simulink model "TV_2017_HIL"  (R2016a)
settings: Solver=ode1  StartTime=0.0  StopTime=600  FixedStep=0.001  RelTol=1e-3
PreLoadFcn:
  | HIL_parameters
values from neighbouring files (symbols this model uses):
  battery_voltage = single(530)    [HIL_parameters.m]    (also in HIL_parameters_2018.m; TV_2017_parameters.m; TV_2017_parameters_VD.m)
  car_params = Simulink_Car_params    [HIL_parameters.m]    (also in HIL_parameters_2018.m; TV_2017_parameters.m; TV_2017_parameters_VD.m)
  i_Diff = 16    [HIL_parameters.m]    (also in HIL_parameters_2018.m; TV_2017_parameters.m)
  Kp = 1    [HIL_parameters.m]    (also in HIL_parameters_2018.m; TV_2017_parameters.m; TV_2017_parameters_VD.m)
  motor_data = struct    [HIL_parameters.m]    (also in HIL_parameters_2018.m; TV_2017_parameters.m)
  settings = Simulink_Settings    [HIL_parameters.m]    (also in HIL_parameters_2018.m; TV_2017_parameters.m; TV_2017_parameters_VD.m)
  SpdC_BCC = 0    [HIL_parameters.m]    (also in HIL_parameters_2018.m; TV_2017_parameters.m; TV_2017_parameters_VD.m)
  Speed_Neg_sat = -21    [HIL_parameters.m]    (also in HIL_parameters_2018.m; TV_2017_parameters.m; TV_2017_parameters_VD.m)
  Speed_Pos_sat = 21    [HIL_parameters.m]    (also in HIL_parameters_2018.m; TV_2017_parameters.m; TV_2017_parameters_VD.m)
  SteeringAngleFL = [-23.80 -22.65 -21.50 -20.34 -19.18 -18.03 -16.86 -15.70 -14.53 -13.35 -12.18 -10.99 -9.80 -8.61 -7.40 -6.19 -4.97 -3.75 -2.51 -1.26 0 1.27 2.56 3.85 5.17 6.50 7.84 9.21 10.59 12.00 13.42 14.88 16.36 17.87 19.41 20.99 22.61 24.26 25.97 27.73 29.54]    [CarSetupAnalysis2018.m]    (also in HIL_parameters_2018.m; TV_2017_parameters.m; TV_2017_parameters_VD.m = [-24.129 -22.950 -21.772 -20.593 -19.413 -18.232 -17.050 -15)
  SteeringAngleFR = [-29.54 -27.73 -25.97 -24.26 -22.61 -20.99 -19.41 -17.87 -16.36 -14.88 -13.42 -12.00 -10.59 -9.21 -7.84 -6.50 -5.17 -3.85 -2.56 -1.27 0 1.26 2.51 3.75 4.97 6.19 7.40 8.61 9.80 10.99 12.18 13.35 14.53 15.70 16.86 18.03 19.18 20.34 21.50 22.65 23.80]    [CarSetupAnalysis2018.m]    (also in HIL_parameters_2018.m; TV_2017_parameters.m; TV_2017_parameters_VD.m = [-29.3050 -27.5340 -25.8140 -24.1410 -22.5110 -20.9180 -19.3)
  SteeringWhAngle = [-105 -99.75 -94.5 -89.25 -84 -78.75 -73.5 -68.25 -63 -57.75 -52.5 -47.25 -42 -36.75 -31.5 -26.25 -21.0 -15.75 -10.5 -5.25 0.0 5.25 10.50 15.75 21.00 26.25 31.50 36.75 42.00 47.25 52.50 57.75  63.00 68.25 73.50 78.75 84.00 89.25 94.50 99.75 105.00]    [TV_2017_parameters_VD.m]
  Tn_n = 0    [HIL_parameters.m]    (also in HIL_parameters_2018.m; TV_2017_parameters.m; TV_2017_parameters_VD.m)
  Use_Joystick = 1    [HIL_parameters.m]    (also in HIL_parameters_2018.m; TV_2017_parameters.m; TV_2017_parameters_VD.m)
undefined symbols (not defined in the file or in its folder): canChannel, TC_Decr_Gas, TC_Derivative, TC_Incr_Gas, TC_On, TC_Relay_Off, TC_Relay_On
libraries: CarMaker4SL x314, canmsglib x48, simulink_extras x48, simulink x41, canlib x39, powerlib_meascontrol x2, sldrtlib x1
(part 1 of 9)
settings Model: Creator=fh  LastModifiedBy=95fre
settings SolverCC: EnableConcurrentExecution=on  InsertRTBMode=Always
settings DataIOCC: LimitDataPoints=on  SaveFormat=Array  SignalLoggingSaveFormat=ModelDataLogs  SignalLoggingName=sigsOut
settings OptimizationCC: BlockReduction=off  OptimizeBlockIOStorage=off  BufferReuse=off  GlobalBufferReuse=off  ExpressionFolding=off  ExpressionDepthLimit=2147483647  LocalBlockOutputs=off  InitFltsAndDblsToZero=on
settings DebuggingCC: SaveWithParameterizedLinksMsg=none  UnderspecifiedInitializationDetection=Classic  MergeDetectMultiDrivingBlocksExec=none  SignalResolutionControl=TryResolveAllWithWarning  MultiTaskDSMMsg=warning  MultiTaskCondExecSysMsg=none  FcnCallInpInsideContextMsg=UseLocalSettings  BusObjectLabelMismatch=error  StateNameClashWarn=warning
settings HardwareCC: ProdBitPerLong=64  ProdLargestAtomicFloat=None  ProdHWDeviceType=Intel->x86-64  TargetBitPerLong=64  TargetBitPerPointer=64  TargetIntDivRoundTo=Zero  TargetEndianess=LittleEndian  TargetWordSize=64  TargetHWDeviceType=Intel->x86-64
settings ModelReferenceCC: PropagateSignalLabelsOutOfModel=off
settings SFSimCC: SimCtrlC=off
settings RTWCC: SystemTargetFile=sldrt.tlc  TemplateMakefile=sldrt.tmf  Description=Simulink Desktop Real-Time  Toolchain=LCC-win64 v2.4.1 | gmake (64-bit Windows)  BuildConfiguration=Faster Runs  RTWCompilerOptimization=on  CheckMdlBeforeBuild=Warning
settings CodeAppCC: MaxIdLength=95
settings SimulinkDesktopRealTimeCC: TargetPreCompLibLocation=C:\Program Files\MATLAB\R2016a\toolbox\sldrt\lib\win64  TargetLangStandard=C89/C90 (ANSI)  SupportVariableSizeSignals=off
settings ConfigComp: CovModelRefEnable=Off

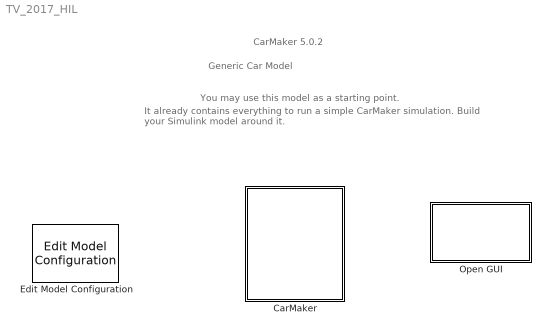
== system TV_2017_HIL ==
  note: Generic Car Model
  note: You may use this model as a starting point.
  note: It already contains everything to run a simple CarMaker simulation.
      | Build your Simulink model around it.
  note: CarMaker 5.0.2
  CarMaker : Subsystem  TreatAsAtomicUnit=on
      mask Display: image(imread('CarMaker4SLss.bmp'));
  Edit Model Configuration : CarMaker4SL/Edit Model Configuration
  Open GUI : Subsystem  LoadFcn=if ~length(which('cmcmd')), cmenv; end
      settings: OpenFcn=cmblockmagic('gui_fix_display'); CM_Simulink
      mask Display: image(imread('CarMakerGUI.bmp'));

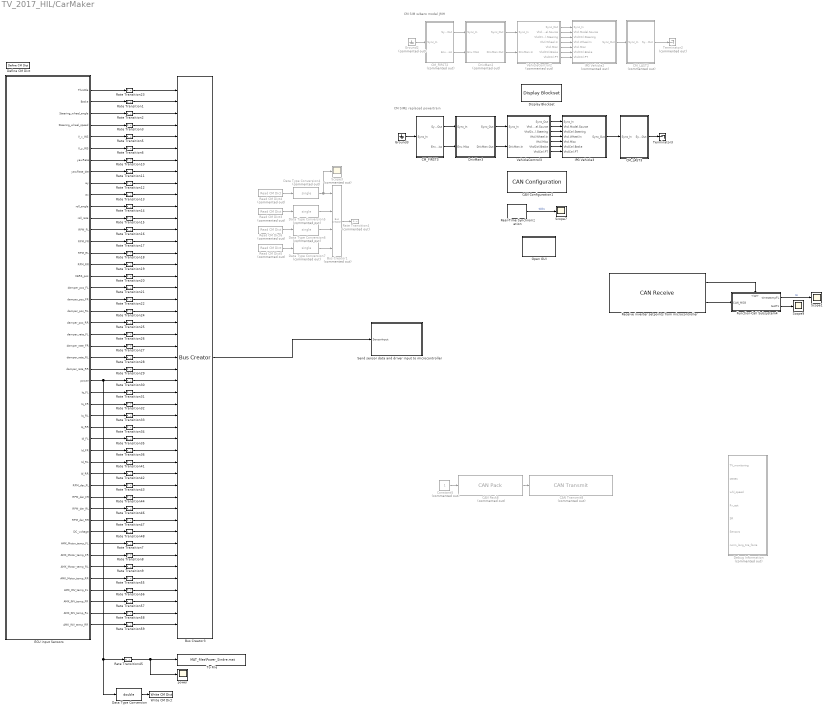
== system TV_2017_HIL/CarMaker ==
  note: CM SIM w/Aero model JMH
  note: CM SIM|| replaced powertrain
  Bus Creator1 : BusCreator  Commented=on  Inputs=4  OutDataTypeStr=Bus: normalForces  NonVirtualBus=on
      settings: InheritFromInputs=off
  Bus Creator3 : BusCreator  Inputs=47  OutDataTypeStr=Bus: SensorInputs  NonVirtualBus=on
      settings: InheritFromInputs=off
  CAN Configuration1 : canlib/CAN Configuration  BlockHandle=8130.0005  DeviceMenu=(none)  Device=PEAK-System PCAN-PCI Express (PCAN_PCIBUS1)  ObjConstructor=canChannel('PEAK-System', 'PCAN_PCIBUS1')  BusSpeed=1000000  EnableBitParameters=off  SJW=NaN  TSEG1=NaN  TSEG2=NaN  NSamples=NaN  AckMode=Normal
  CAN Pack8 : canmsglib/CAN Pack  Commented=on  MsgList=(none)  MsgName=CAN Msg  MsgIDType=Standard (11-bit identifier)  MsgIdentifier=5  MsgLength=1  SignalInfo=Signal1$0$8$1$1$1$0$1$0$-Inf$Inf$#  NSignals=1  StartBits=str2num('[int32(0)]')  SignalSizes=str2num('[int32(8)]')  ByteOrders=str2num('[int32(1)]')  DataTypes=str2num('[int32(1)]')  MultiplexTypes=str2num('[int32(1)]')  MultiplexValues=str2num('[double(0)]')  Factors=str2num('[double(1)]')  Offsets=str2num('[double(0)]')  Minimums=str2num('[double(-Inf)]')  Maximums=str2num('[double(Inf)]')  Remote=off
      settings: DataFormat=manually specified signals
  CAN Transmit8 : canlib/CAN Transmit  Commented=on  BlockHandle=8132.0005  DeviceMenu=(none)  Device=PEAK-System PCAN-PCI Express (PCAN_PCIBUS1)  ObjConstructor=canChannel('PEAK-System', 'PCAN_PCIBUS1')  EnablePeriodicTransmit=off  MessagePeriod=1.000
  CM_FIRST2 : Subsystem  Commented=on
  CM_FIRST3 : Subsystem
  CM_LAST2 : Subsystem  Commented=on
  CM_LAST3 : Subsystem
  Constant5 : Constant  Commented=on
  Data Type Conversion : DataTypeConversion  OutDataTypeStr=double
  Data Type Conversion{4..7} (4 alike) : DataTypeConversion  Commented=on  OutDataTypeStr=single
  "Debug Information " : Subsystem  Commented=on
  Define CM Dict : CarMaker4SL/Define CM Dict  xname=Power  xmono=off  xtype=Double  xdvaplace=None  xnstates=0  xfirststate=0  xinitial=0
  Display Blockset : CarMaker4SL/Display Blockset
  DrivMan2 : Subsystem  Commented=on
  DrivMan3 : Subsystem
  "ECU input Sensors " : Subsystem  SystemSampleTime=settings.control_system_sample_time
  Function-Call Subsystem4 : Subsystem  TreatAsAtomicUnit=on
  Ground2 : Ground  Commented=on
  Ground3 : Ground
  IPG Vehicle2 : Subsystem  Commented=on  TreatAsAtomicUnit=on
  IPG Vehicle3 : Subsystem  TreatAsAtomicUnit=on
  Open GUI : Subsystem  LoadFcn=if ~length(which('cmcmd')), cmenv; end
      settings: OpenFcn=cmblockmagic('gui_fix_display'); CM_Simulink
      mask Display: image(imread('CarMakerGUI.bmp'));
  Rate Transition{1..3,5..36,41..48,55..59} (48 alike) : RateTransition  OutPortSampleTime=matlab_params.sensor_sampling_time
  Rate Transition4 : RateTransition  Commented=on  OutPortSampleTime=settings.sensor_sampling_time
  Read CM Dict3 : CarMaker4SL/Read CM Dict  Commented=on  xname=Vhcl.FR.Fz  xsync=off
  Read CM Dict4 : CarMaker4SL/Read CM Dict  Commented=on  xname=Vhcl.FL.Fz  xsync=off
  Read CM Dict5 : CarMaker4SL/Read CM Dict  Commented=on  xname=Vhcl.RR.Fz  xsync=off
  Read CM Dict6 : CarMaker4SL/Read CM Dict  Commented=on  xname=Vhcl.RL.Fz  xsync=off
  Real-Time Synchronization : sldrtlib/Real-Time Synchronization  SampleTime=0.01  MaxMissedTicks=100000  ShowMissedTicks=on  YieldWhenWaiting=on
  Receive inverter setpoints from microcontroller : canlib/CAN Receive  BlockHandle=21848.0001  DeviceMenu=(none)  Device=PEAK-System PCAN-PCI Express (PCAN_PCIBUS1)  ObjConstructor=canChannel('PEAK-System', 'PCAN_PCIBUS1')  EnableStandardIDsFilter=off  StandardIDs=listen_ID  EnableExtendedIDsFilter=off  ExtendedIDs=0  SampleTime=0.001  MsgsPerTimestep=all  StdIDsCombo=Allow all  ExtIDsCombo=Block all  InternalFilterUpdateStatus=on
  Scope1 : Scope
  Scope3 : Scope  Commented=on
  Scope7 : Scope
  Scope9 : Scope
  "Send sensor data and driver input to microcontroller " : Subsystem
  Terminator2 : Terminator  Commented=on
  Terminator3 : Terminator
  To File : ToFile  Filename=MAT_files\Power_Sindre.mat  MatrixName=Power  SaveFormat=Timeseries
  VehicleControl2 : Subsystem  Commented=on
  VehicleControl3 : Subsystem
  Write CM Dict : CarMaker4SL/Write CM Dict  xname=Power  xsync=off
  power : Scope
  wires:
  Read CM Dict3/1 -> Data Type Conversion5/1
  Read CM Dict4/1 -> Data Type Conversion4/1
  Read CM Dict5/1 -> Data Type Conversion7/1
  Read CM Dict6/1 -> Data Type Conversion6/1
  Data Type Conversion6/1 -> Bus Creator1/3
  Data Type Conversion7/1 -> Bus Creator1/4
  Data Type Conversion5/1 -> Bus Creator1/2
  Data Type Conversion4/1 -> Scope3/1, Bus Creator1/1
  Bus Creator1/1 -> Rate Transition4/1
  Real-Time Synchronization/1 -> Scope7/1  "ticks"
  Receive inverter setpoints from microcontroller/2 -> Function-Call Subsystem4/1(CAN_MSG)
  Receive inverter setpoints from microcontroller/1 -> Function-Call Subsystem4/Trigger
  Function-Call Subsystem4/1(timestampFL) -> Scope1/1  "ts"
  Function-Call Subsystem4/2(testTs) -> Scope9/1
  ? -> ?
  CAN Pack8/1 -> CAN Transmit8/1
  Constant5/1 -> CAN Pack8/1
  CM_FIRST2/2(Env.Misc) -> DrivMan2/2(Env.Misc)
  VehicleControl2/2(Vhcl.Model.Source) -> IPG Vehicle2/2(Vhcl.Model.Source)
  VehicleControl2/6(VhclCtrl.Brake) -> IPG Vehicle2/6(VhclCtrl.Brake)
  VehicleControl2/3(VhclCtrl.Steering) -> IPG Vehicle2/3(VhclCtrl.Steering)
  DrivMan2/2(DrivMan.Out) -> VehicleControl2/2(DrivMan.In)
  CM_FIRST2/1(Sync_Out) -> DrivMan2/1(Sync_In)
  VehicleControl2/7(VhclCtrl.PT) -> IPG Vehicle2/7(VhclCtrl.PT)
  VehicleControl2/4(Vhcl.Wheel.In) -> IPG Vehicle2/4(Vhcl.Wheel.In)
  VehicleControl2/1(Sync_Out) -> IPG Vehicle2/1(Sync_In)
  IPG Vehicle2/1(Sync_Out) -> CM_LAST2/1(Sync_In)
  DrivMan2/1(Sync_Out) -> VehicleControl2/1(Sync_In)
  Ground2/1 -> CM_FIRST2/1(Sync_In)
  CM_LAST2/1(Sync_Out) -> Terminator2/1
  VehicleControl2/5(Vhcl.Misc) -> IPG Vehicle2/5(Vhcl.Misc)
  VehicleControl3/7(VhclCtrl.PT) -> IPG Vehicle3/7(VhclCtrl.PT)
  VehicleControl3/6(VhclCtrl.Brake) -> IPG Vehicle3/6(VhclCtrl.Brake)
  CM_FIRST3/1(Sync_Out) -> DrivMan3/1(Sync_In)
  CM_FIRST3/2(Env.Misc) -> DrivMan3/2(Env.Misc)
  VehicleControl3/3(VhclCtrl.Steering) -> IPG Vehicle3/3(VhclCtrl.Steering)
  DrivMan3/2(DrivMan.Out) -> VehicleControl3/2(DrivMan.In)
  VehicleControl3/2(Vhcl.Model.Source) -> IPG Vehicle3/2(Vhcl.Model.Source)
  VehicleControl3/5(Vhcl.Misc) -> IPG Vehicle3/5(Vhcl.Misc)
  VehicleControl3/1(Sync_Out) -> IPG Vehicle3/1(Sync_In)
  VehicleControl3/4(Vhcl.Wheel.In) -> IPG Vehicle3/4(Vhcl.Wheel.In)
  DrivMan3/1(Sync_Out) -> VehicleControl3/1(Sync_In)
  Ground3/1 -> CM_FIRST3/1(Sync_In)
  IPG Vehicle3/1(Sync_Out) -> CM_LAST3/1(Sync_In)
  CM_LAST3/1(Sync_Out) -> Terminator3/1
  Rate Transition45/1 -> power/1, To File/1
  "ECU input Sensors "/37(RPM_der_RL) -> Rate Transition46/1
  "ECU input Sensors "/38(RPM_der_RR) -> Rate Transition47/1
  "ECU input Sensors "/36(RPM_der_FR) -> Rate Transition44/1
  "ECU input Sensors "/35(RPM_der_FL) -> Rate Transition43/1
  "ECU input Sensors "/34(Id_RR) -> Rate Transition42/1
  "ECU input Sensors "/4(Steering_wheel_speed) -> Rate Transition3/1
  "ECU input Sensors "/1("Throttle ") -> Rate Transition23/1
  "ECU input Sensors "/2("Brake ") -> Rate Transition1/1
  "ECU input Sensors "/3("Steering_wheel_angle ") -> Rate Transition2/1
  "ECU input Sensors "/5(V_x_INS) -> Rate Transition5/1
  "ECU input Sensors "/6(V_y_INS) -> Rate Transition6/1
  "ECU input Sensors "/7(yawRate) -> Rate Transition10/1
  "ECU input Sensors "/9(ay) -> Rate Transition12/1
  "ECU input Sensors "/10("ax ") -> Rate Transition13/1
  "ECU input Sensors "/11(roll_angle) -> Rate Transition14/1
  "ECU input Sensors "/12(roll_rate) -> Rate Transition15/1
  "ECU input Sensors "/13(RPM_FL) -> Rate Transition16/1
  "ECU input Sensors "/14(RPM_FR) -> Rate Transition17/1
  "ECU input Sensors "/15(RPM_RL) -> Rate Transition18/1
  "ECU input Sensors "/16(RPM_RR) -> Rate Transition19/1
  "ECU input Sensors "/17(KERS_pos) -> Rate Transition20/1
  "ECU input Sensors "/18(damper_pos_FL) -> Rate Transition21/1
  "ECU input Sensors "/19(damper_pos_FR) -> Rate Transition22/1
  "ECU input Sensors "/20(damper_pos_RL) -> Rate Transition24/1
  "ECU input Sensors "/21(damper_pos_RR) -> Rate Transition25/1
  "ECU input Sensors "/22(damper_rate_FL) -> Rate Transition26/1
  "ECU input Sensors "/23(damper_rate_FR) -> Rate Transition27/1
  "ECU input Sensors "/24(damper_rate_RL) -> Rate Transition28/1
  "ECU input Sensors "/25(damper_rate_RR) -> Rate Transition29/1
  "ECU input Sensors "/27(Iq_FL) -> Rate Transition31/1
  "ECU input Sensors "/28(Iq_FR) -> Rate Transition32/1
  "ECU input Sensors "/29(Iq_RL) -> Rate Transition33/1
  "ECU input Sensors "/30(Iq_RR) -> Rate Transition34/1
  "ECU input Sensors "/31(Id_FL) -> Rate Transition35/1
  "ECU input Sensors "/32(Id_FR) -> Rate Transition36/1
  "ECU input Sensors "/33(Id_RL) -> Rate Transition41/1
  "ECU input Sensors "/8(yawRate_der) -> Rate Transition11/1
  "ECU input Sensors "/39(DC_voltage) -> Rate Transition48/1
  Rate Transition23/1 -> Bus Creator3/1
  Rate Transition17/1 -> Bus Creator3/14
  Rate Transition12/1 -> Bus Creator3/9
  Rate Transition30/1 -> Bus Creator3/26
  Rate Transition14/1 -> Bus Creator3/11
  Rate Transition16/1 -> Bus Creator3/13
  Rate Transition25/1 -> Bus Creator3/21
  Rate Transition3/1 -> Bus Creator3/4
  Rate Transition2/1 -> Bus Creator3/3
  Rate Transition22/1 -> Bus Creator3/19
  Rate Transition11/1 -> Bus Creator3/8
  Rate Transition18/1 -> Bus Creator3/15
  Rate Transition20/1 -> Bus Creator3/17
  Rate Transition1/1 -> Bus Creator3/2
  Rate Transition24/1 -> Bus Creator3/20
  Rate Transition31/1 -> Bus Creator3/27
  Rate Transition26/1 -> Bus Creator3/22
  Rate Transition29/1 -> Bus Creator3/25
  Rate Transition15/1 -> Bus Creator3/12
  Rate Transition13/1 -> Bus Creator3/10
  Rate Transition28/1 -> Bus Creator3/24
  Rate Transition19/1 -> Bus Creator3/16
  Rate Transition21/1 -> Bus Creator3/18
  Rate Transition27/1 -> Bus Creator3/23
  Rate Transition5/1 -> Bus Creator3/5
  Rate Transition6/1 -> Bus Creator3/6
  Rate Transition42/1 -> Bus Creator3/34
  Rate Transition47/1 -> Bus Creator3/38
  Rate Transition48/1 -> Bus Creator3/39
  Rate Transition41/1 -> Bus Creator3/33
  Rate Transition43/1 -> Bus Creator3/35
  Rate Transition35/1 -> Bus Creator3/31
  Rate Transition34/1 -> Bus Creator3/30
  Rate Transition46/1 -> Bus Creator3/37
  Rate Transition44/1 -> Bus Creator3/36
  Rate Transition33/1 -> Bus Creator3/29
  Rate Transition32/1 -> Bus Creator3/28
  Rate Transition36/1 -> Bus Creator3/32
  Rate Transition10/1 -> Bus Creator3/7
  "ECU input Sensors "/26(power) -> Data Type Conversion/1, Rate Transition45/1, Rate Transition30/1
  Data Type Conversion/1 -> Write CM Dict/1
  "ECU input Sensors "/44(AMK_INV_temp_FL) -> Rate Transition56/1
  "ECU input Sensors "/40(AMK_Motor_temp_FL) -> Rate Transition7/1
  "ECU input Sensors "/41(AMK_Motor_temp_FR) -> Rate Transition8/1
  "ECU input Sensors "/42(AMK_Motor_temp_RL) -> Rate Transition9/1
  "ECU input Sensors "/43(AMK_Motor_temp_RR) -> Rate Transition55/1
  "ECU input Sensors "/45(AMK_INV_temp_FR) -> Rate Transition57/1
  "ECU input Sensors "/46(AMK_INV_temp_RL) -> Rate Transition58/1
  "ECU input Sensors "/47(AMK_INV_temp_RR) -> Rate Transition59/1
  Rate Transition7/1 -> Bus Creator3/40
  Rate Transition8/1 -> Bus Creator3/41
  Rate Transition9/1 -> Bus Creator3/42
  Rate Transition55/1 -> Bus Creator3/43
  Rate Transition56/1 -> Bus Creator3/44
  Rate Transition57/1 -> Bus Creator3/45
  Rate Transition58/1 -> Bus Creator3/46
  Rate Transition59/1 -> Bus Creator3/47
  Bus Creator3/1 -> "Send sensor data and driver input to microcontroller "/1(SensorInput)

== system TV_2017_HIL/Open GUI ==
  S-Function : S-Function  FunctionName=cm_gui  SFunctionDeploymentMode=off  EnableBusSupport=off

== system TV_2017_HIL/CarMaker/CM_FIRST2 ==
  Sync_In : Inport
  Bus Creator1 : BusCreator  Inputs=9
  Demux : Demux  Outputs=9
  Environment : S-Function  FunctionName=CM_Sfun  Parameters='Environment'  SFunctionDeploymentMode=off  EnableBusSupport=off
  IoIn : S-Function  FunctionName=CM_Sfun  Parameters='IoIn'  SFunctionDeploymentMode=off  EnableBusSupport=off
  Sync_Out : Outport
  Env.Misc : Outport  Port=2
  wires:
  Bus Creator1/1 -> Env.Misc/1
  Environment/2 -> Demux/1
  Demux/4 -> Bus Creator1/4  "Env AirHumidity"
  Demux/3 -> Bus Creator1/3  "Env AirPressure"
  Demux/2 -> Bus Creator1/2  "Env AirDensity"
  Demux/1 -> Bus Creator1/1  "Env Temperature"
  Environment/1 -> Sync_Out/1
  IoIn/1 -> Environment/1
  Sync_In/1 -> IoIn/1
  Demux/5 -> Bus Creator1/5  "Env Time"
  Demux/6 -> Bus Creator1/6  "Env SolarRadiation"
  Demux/7 -> Bus Creator1/7  "Env WindVel_tot x"
  Demux/8 -> Bus Creator1/8  "Env WindVel_tot y"
  Demux/9 -> Bus Creator1/9  "Env WindVel_tot z"

== system TV_2017_HIL/CarMaker/CM_FIRST3 ==
  Sync_In : Inport
  BusCreator1 : BusCreator  Inputs=8
  BusCreator2 : BusCreator  Inputs=6
  Demux1 : Demux  Outputs=14
  Environment : S-Function  FunctionName=CM_Sfun  Parameters='Environment'  SFunctionDeploymentMode=off  EnableBusSupport=off
  IoIn : S-Function  FunctionName=CM_Sfun  Parameters='IoIn'  SFunctionDeploymentMode=off  EnableBusSupport=off
  Terminator : Terminator
  Sync_Out : Outport
  Env.Misc : Outport  Port=2
  wires:
  BusCreator2/1 -> Terminator/1  "IF Environment (in)"
  BusCreator1/1 -> Env.Misc/1
  Demux1/14 -> BusCreator2/6  "Env sRoad"
  Demux1/13 -> BusCreator2/5  "Env PoI_GCS Elev"
  Demux1/12 -> BusCreator2/4  "Env PoI_GCS Lat"
  Demux1/11 -> BusCreator2/3  "Env PoI_GCS Long"
  Demux1/10 -> BusCreator2/2  "Env Time"
  Demux1/9 -> BusCreator2/1  "Env yDay"
  Demux1/8 -> BusCreator1/8  "Env WindVel_tot z"
  Demux1/7 -> BusCreator1/7  "Env WindVel_tot y"
  Demux1/6 -> BusCreator1/6  "Env WindVel_tot x"
  Demux1/5 -> BusCreator1/5  "Env SolarRadiation"
  Demux1/4 -> BusCreator1/4  "Env AirHumidity"
  Demux1/3 -> BusCreator1/3  "Env AirPressure"
  Demux1/2 -> BusCreator1/2  "Env AirDensity"
  Demux1/1 -> BusCreator1/1  "Env Temperature"
  Environment/2 -> Demux1/1
  Environment/1 -> Sync_Out/1
  IoIn/1 -> Environment/1
  Sync_In/1 -> IoIn/1

== system TV_2017_HIL/CarMaker/CM_LAST2 ==
  Sync_In : Inport
  CM_User : S-Function  FunctionName=CM_Sfun  Parameters='CM_User'  SFunctionDeploymentMode=off  EnableBusSupport=off
  IoOut : S-Function  FunctionName=CM_Sfun  Parameters='IoOut'  SFunctionDeploymentMode=off  EnableBusSupport=off
  Sync_Out : Outport
  wires:
  IoOut/1 -> Sync_Out/1
  CM_User/1 -> IoOut/1
  Sync_In/1 -> CM_User/1

== system TV_2017_HIL/CarMaker/CM_LAST3 ==
  Sync_In : Inport
  CM_User : S-Function  FunctionName=CM_Sfun  Parameters='CM_User'  SFunctionDeploymentMode=off  EnableBusSupport=off
  IoOut : S-Function  FunctionName=CM_Sfun  Parameters='IoOut'  SFunctionDeploymentMode=off  EnableBusSupport=off
  Sync_Out : Outport
  wires:
  IoOut/1 -> Sync_Out/1
  CM_User/1 -> IoOut/1
  Sync_In/1 -> CM_User/1

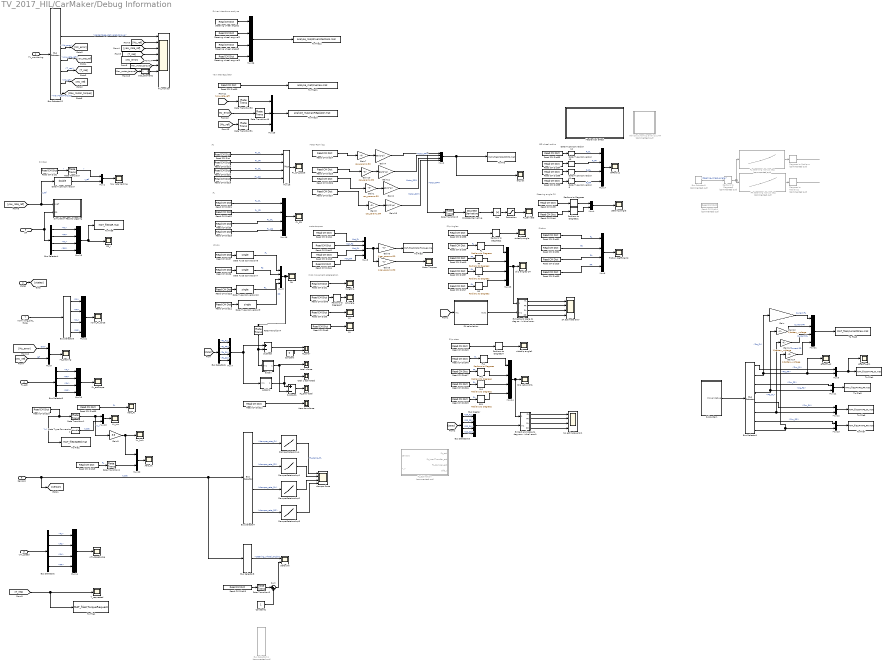
== system TV_2017_HIL/CarMaker/Debug Information  ==
  note: SimRes
  note: Eff wheel radius
  note: motortorques
  note: Friction
  note: FZ CM
  note: Fy
  note: FX
  note: misc movement acceleration
  note: Steering angle CM
  note: Motor Rpm log
  note: Slip Angles
  note: Slip rates
  note: Yaw rate regulator
  note: Driver intentions analyze
  TV_monitoring : Inport
  states : Inport  Port=2
  whl_speed : Inport  Port=3
  Fx_est : Inport  Port=4
  "SR " : Inport  Port=5
  Sensors : Inport  Port=6
  norm_long_tire_force : Inport  Port=7
  Abs : Abs
  "Aero downforce " : Scope
  Aero_Fx : Scope
  Aero_Fz : Scope
  Bus Creator : BusCreator  Inputs=4
  Bus Selector1 : BusSelector  OutputSignals=Pm_FL,Pe_FL,Pm_FR,Pe_FR,Pm_RL,Pe_RL,Pm_RR,Pe_RR
  Bus Selector10 : BusSelector  OutputSignals=SR_FL,SR_FR,SR_RL,SR_RR
  Bus Selector11 : BusSelector  Commented=on  OutputSignals=steering_wheel_angle
  Bus Selector12 : BusSelector  OutputSignals=active_contraints,saturated_constraints,percentage_delivered_torque,Mz_error,yaw_rate_ref,T_req,Mz_ref,maxMotorTorque
  Bus Selector{2..5} (4 alike) : BusSelector  OutputSignals=FL,FR,RL,RR
  Bus Selector6 : BusSelector  OutputSignals=Fz_FL,Fz_FR,Fz_RL,Fz_RR
  Bus Selector7 : BusSelector  OutputSignals=damper_rate_FL,damper_rate_FR,damper_rate_RL,damper_rate_RR
  Bus Selector8 : BusSelector  OutputSignals=steering_wheel_angle
  Bus Selector9 : BusSelector  Commented=on  OutputSignals=steering_wheel_angle
  Constant : Constant  Value=0
  Constant1 : Constant
  DamperRateLookup : Lookup_n-D  NumberOfTableDimensions=1  BreakpointsForDimension1=car_params.damper_table_breakpoint;  Table=car_params.damper_pull_push_values_front;  ExtrapMethod=Clip  UseLastTableValue=on  InternalRulePriority=Speed  RndMeth=Simplest  InputSameDT=on
  DamperRateLookup1 : Lookup_n-D  NumberOfTableDimensions=1  BreakpointsForDimension1=car_params.damper_table_breakpoint;  Table=car_params.damper_pull_push_values_front;  ExtrapMethod=Clip  UseLastTableValue=on  InternalRulePriority=Speed  RndMeth=Simplest  InputSameDT=on
  DamperRateLookup2 : Lookup_n-D  NumberOfTableDimensions=1  BreakpointsForDimension1=car_params.damper_table_breakpoint;  Table=car_params.damper_pull_push_values_rear;  ExtrapMethod=Clip  UseLastTableValue=on  InternalRulePriority=Speed  RndMeth=Simplest  InputSameDT=on
  DamperRateLookup3 : Lookup_n-D  NumberOfTableDimensions=1  BreakpointsForDimension1=car_params.damper_table_breakpoint;  Table=car_params.damper_pull_push_values_rear;  ExtrapMethod=Clip  UseLastTableValue=on  InternalRulePriority=Speed  RndMeth=Simplest  InputSameDT=on
  Data Type Conversion : DataTypeConversion  OutDataTypeStr=double
  Data Type Conversion1 : DataTypeConversion  OutDataTypeStr=double
  Data Type Conversion{6..13} (8 alike) : DataTypeConversion  OutDataTypeStr=single
  Degrees to Radians : simulink_extras/Transformations/Degrees to Radians  Commented=on
  Degrees to Radians1 : simulink_extras/Transformations/Degrees to Radians  Commented=on
  Discrete Derivative : simulink/Discrete/Discrete Derivative  gainval=1.0  ICPrevScaledInput=0.0  InputProcessing=Inherited  OutMin=[]  OutMax=[]  OutDataType=fixdt(1, 16)  OutScaling=2^-10  DoSatur=off
  Extract and scale to deg compare to CM output in individual error : Subsystem
  Extract and scale to deg compare to CM output in individual error1 : Subsystem
  FL : simulink_extras/Transformations/Radians to Degrees
  FL steer ang lookup deg : Lookup_n-D  Commented=on  NumberOfTableDimensions=1  BreakpointsForDimension1=SteeringWhAngle  Table=SteeringAngleFL  ExtrapMethod=Clip  UseLastTableValue=on  InternalRulePriority=Speed  RndMeth=Simplest  InputSameDT=on
  FL1 : simulink_extras/Transformations/Radians to Degrees
  FR : simulink_extras/Transformations/Radians to Degrees
  FR steer ang lookup deg : Lookup_n-D  Commented=on  NumberOfTableDimensions=1  BreakpointsForDimension1=SteeringWhAngle  Table=SteeringAngleFR  ExtrapMethod=Clip  UseLastTableValue=on  InternalRulePriority=Speed  RndMeth=Simplest  InputSameDT=on
  FR1 : simulink_extras/Transformations/Radians to Degrees
  FY_CM : Scope
  Fl_derivate : Scope
  Fx_CM_scope : Scope
  Fx_estScope : Scope
  Fz_Estimation : Subsystem  Commented=on  TreatAsAtomicUnit=on
  Fz_error : Scope  NumInputPorts=2
  Fz_error total : Scope
  Fzi : Scope
  Gain{,12..14} (4 alike) : Gain  Gain=1/battery_voltage
  Gain{1,3,7,10} (4 alike) : Gain  Gain=car_params.GR
  Gain{2,4,11,15} (4 alike) : Gain  Gain=60/(2*pi)
  Gain5 : Gain  Gain=1/car_params.GR
  Gain6 : Gain  Gain=1/car_params.GR
  Gain9 : Gain  Gain=3.6
  Mechanical effect : Subsystem
  "Motor Torques " : Scope
  Mux{1,4..5,9..13,20} (9 alike) : Mux  Inputs=2
  Mux{2..3,6..8,14..19,21..24,26} (16 alike) : Mux
  Mux25 : Mux  Inputs=3
  Mz_tracking : Scope
  RL : simulink_extras/Transformations/Radians to Degrees
  RL1 : simulink_extras/Transformations/Radians to Degrees
  RR : simulink_extras/Transformations/Radians to Degrees
  RR1 : simulink_extras/Transformations/Radians to Degrees
  Radians to Degrees{,1..2,4,7} (5 alike) : simulink_extras/Transformations/Radians to Degrees
  Radians to Degrees3 : simulink_extras/Transformations/Radians to Degrees  Commented=on
  Rate Transition{,1..5} (6 alike) : RateTransition  OutPortSampleTime=matlab_params.control_system_sample_time
  Rate Transition49 : RateTransition  OutPortSampleTimeOpt=Inherit
  Rate Transition50 : RateTransition  OutPortSampleTimeOpt=Inherit
  Rate Transition51 : RateTransition  OutPortSampleTimeOpt=Inherit
  Read CM Dict : CarMaker4SL/Read CM Dict  xname=Vhcl.FL.Fx  xsync=off
  Read CM Dict1 : CarMaker4SL/Read CM Dict  xname=Car.LongSlipRL  xsync=off
  Read CM Dict10 : CarMaker4SL/Read CM Dict  xname=Car.vx  xsync=off
  Read CM Dict11 : CarMaker4SL/Read CM Dict  xname=Vhcl.RR.Fz  xsync=off
  Read CM Dict12 : CarMaker4SL/Read CM Dict  xname=Car.Aero.Frc_1.z  xsync=off
  Read CM Dict13 : CarMaker4SL/Read CM Dict  xname=Vhcl.Steer.Ang  xsync=off
  Read CM Dict14 : CarMaker4SL/Read CM Dict  Commented=on  xsync=off
  Read CM Dict15 : CarMaker4SL/Read CM Dict  xname=Car.LongSlipRR  xsync=off
  Read CM Dict16 : CarMaker4SL/Read CM Dict  xname=Car.LongSlipRL  xsync=off
  Read CM Dict17 : CarMaker4SL/Read CM Dict  xname=Car.SlipAngleRR  xsync=off
  Read CM Dict18 : CarMaker4SL/Read CM Dict  xname=Vhcl.FR.Fx  xsync=off
  Read CM Dict19 : CarMaker4SL/Read CM Dict  xname=Vhcl.RR.Fx  xsync=off
  Read CM Dict2 : CarMaker4SL/Read CM Dict  xname=Car.YawRate  xsync=off
  Read CM Dict20 : CarMaker4SL/Read CM Dict  xname=Vhcl.RL.Fx  xsync=off
  Read CM Dict21 : CarMaker4SL/Read CM Dict  xname=Vhcl.FL.Fy  xsync=off
  Read CM Dict22 : CarMaker4SL/Read CM Dict  xname=Vhcl.FR.Fy  xsync=off
  Read CM Dict23 : CarMaker4SL/Read CM Dict  xname=Vhcl.RR.Fy  xsync=off
  Read CM Dict24 : CarMaker4SL/Read CM Dict  xname=Car.WheelSpd_FL  xsync=off
  Read CM Dict25 : CarMaker4SL/Read CM Dict  xname=Car.WheelSpd_FR  xsync=off
  Read CM Dict26 : CarMaker4SL/Read CM Dict  xname=Car.WheelSpd_RL  xsync=off
  Read CM Dict27 : CarMaker4SL/Read CM Dict  xname=Car.WheelSpd_RR  xsync=off
  Read CM Dict28 : CarMaker4SL/Read CM Dict  xname=Vhcl.RL.Fz  xsync=off
  Read CM Dict29 : CarMaker4SL/Read CM Dict  xname=Car.muRoadRL  xsync=off
  Read CM Dict3 : CarMaker4SL/Read CM Dict  xname=Car.CFR.rz  xsync=off
  Read CM Dict30 : CarMaker4SL/Read CM Dict  xname=Car.muRoadRR  xsync=off
  Read CM Dict31 : CarMaker4SL/Read CM Dict  xname=Car.muRoadFL  xsync=off
  Read CM Dict32 : CarMaker4SL/Read CM Dict  xname=Car.muRoadFR  xsync=off
  Read CM Dict33 : CarMaker4SL/Read CM Dict  xname=Car.WFL.Radius  xsync=off
  Read CM Dict34 : CarMaker4SL/Read CM Dict  xname=Car.WFR.Radius  xsync=off
  Read CM Dict35 : CarMaker4SL/Read CM Dict  xname=Car.WRR.Radius  xsync=off
  Read CM Dict36 : CarMaker4SL/Read CM Dict  xname=Car.WRL.Radius  xsync=off
  Read CM Dict37 : CarMaker4SL/Read CM Dict  xname=Car.SlipAngleRL  xsync=off
  Read CM Dict38 : CarMaker4SL/Read CM Dict  xname=Car.SideSlipAngle  xsync=off
  Read CM Dict39 : CarMaker4SL/Read CM Dict  xname=Car.SlipAngleFL  xsync=off
  Read CM Dict4 : CarMaker4SL/Read CM Dict  xname=Car.CFL.rz  xsync=off
  Read CM Dict40 : CarMaker4SL/Read CM Dict  xname=Car.SlipAngleFR  xsync=off
  Read CM Dict41 : CarMaker4SL/Read CM Dict  xname=PT.WFL.Trq_Drive  xsync=off
  Read CM Dict42 : CarMaker4SL/Read CM Dict  xname=PT.WFR.Trq_Drive  xsync=off
  Read CM Dict43 : CarMaker4SL/Read CM Dict  xname=PT.WRL.Trq_Drive  xsync=off
  Read CM Dict44 : CarMaker4SL/Read CM Dict  xname=PT.WRR.Trq_Drive  xsync=off
  Read CM Dict45 : CarMaker4SL/Read CM Dict  xname=Car.SideSlipAngle  xsync=off
  Read CM Dict46 : CarMaker4SL/Read CM Dict  xname=Car.LongSlipFL  xsync=off
  Read CM Dict47 : CarMaker4SL/Read CM Dict  xname=Car.LongSlipFR  xsync=off
  Read CM Dict48 : CarMaker4SL/Read CM Dict  xname=Vhcl.Roll  xsync=off
  Read CM Dict49 : CarMaker4SL/Read CM Dict  xname=Car.Aero.Frc_1.z  xsync=off
  Read CM Dict5 : CarMaker4SL/Read CM Dict  xname=Vhcl.RL.Fy  xsync=off
  Read CM Dict50 : CarMaker4SL/Read CM Dict  xname=Vhcl.YawRate  xsync=off
  Read CM Dict53 : CarMaker4SL/Read CM Dict  xname=Car.Aero.Frc_1.x  xsync=off
  Read CM Dict6 : CarMaker4SL/Read CM Dict  xname=Vhcl.FR.Fz  xsync=off
  Read CM Dict7 : CarMaker4SL/Read CM Dict  xname=Vhcl.FL.Fz  xsync=off
  Read CM Dict8 : CarMaker4SL/Read CM Dict  xname=Car.ax  xsync=off
  Read CM Dict9 : CarMaker4SL/Read CM Dict  xname=Car.ay  xsync=off
  SA calculation : Subsystem
  SA estimate error : Scope  NumInputPorts=4
  SA estimate error1 : Scope  NumInputPorts=4
  SR_i : Scope
  Saturation : Saturate  UpperLimit=50000
  Simulation Results Logging : Subsystem
  Slip angles CM : Scope
  Slip ratios CM1 : Scope
  Steering wheel ang-vel2 : CarMaker4SL/Read CM Dict  xname=DM.Steer.AngVel  xsync=off
  Steering wheel ang-vel3 : CarMaker4SL/Read CM Dict  xname=DM.Brake  xsync=off
  Steering wheel angle2 : CarMaker4SL/Read CM Dict  xname=DM.Steer.Ang  xsync=off
  Steering wheel angle3 : CarMaker4SL/Read CM Dict  xname=DM.Gas  xsync=off
  Subsystem : Subsystem
  Subtract : Sum  Inputs=+-
  Subtract1 : Sum  Inputs=+-
  Sum : Sum  Inputs=|++
  TV_monitor : Scope  NumInputPorts=9
  "T_requested " : Scope
  To File : ToFile  Filename=MAT_files\MotorRPMS.mat  MatrixName=MotorRpms  SaveFormat=Timeseries
  To File1 : ToFile  Filename=MAT_files\TorqueRequest  MatrixName=TorqueRequest  SaveFormat=Timeseries
  To File10 : ToFile  Filename=analyse_mat/yawRegulator.mat  MatrixName=yaw_reg  SaveFormat=Timeseries
  To File11 : ToFile  Filename=analyse_mat/trueYaw.mat  MatrixName=vhclYaw  SaveFormat=Timeseries
  To File12 : ToFile  Filename=analyse_mat/driverIntentions.mat  MatrixName=driverIntentions  SaveFormat=Timeseries
  To File2 : ToFile  Filename=MAT_files\Speed.mat  MatrixName=VehicleSpeed  SaveFormat=Timeseries
  To File3 : ToFile  Filename=MAT_files\MotorTorques.mat  MatrixName=MotorTorques  SaveFormat=Timeseries
  To File4 : ToFile  Filename=MAT_files\PmPe_FL.mat  MatrixName=PmPe_FL  SaveFormat=Timeseries
  To File5 : ToFile  Filename=MAT_files\PmPe_FR.mat  MatrixName=PmPe_FR  SaveFormat=Timeseries
  To File6 : ToFile  Filename=MAT_files\PmPe_RL.mat  MatrixName=PmPe_RL  SaveFormat=Timeseries
  To File7 : ToFile  Filename=MAT_files\PmPe_RR.mat  MatrixName=PmPe_RR  SaveFormat=Timeseries
  To File8 : ToFile  Filename=MAT_files\SR.mat  MatrixName=SR  SaveFormat=Timeseries
  To File9 : ToFile  Filename=MAT_files\currentDraw.mat  SaveFormat=Timeseries
  Vehicle dynamics analysis JMH : Subsystem  Commented=on
  Vx_kmh : Scope
  "Vx_ms " : Scope
  Yaw rate tracking : Scope
  add_elements : Subsystem
  addall : Subsystem
  addall1 : Subsystem
  ax : Scope
  ay : Scope
  damper force : Scope  NumInputPorts=4
  delta SW : Scope  NumInputPorts=2
  effRadius : Scope
  effectFL_el : Scope
  effectFL_el1 : Scope
  eng rot : Scope
  friction coefficients : Scope
  "longSlip " : Scope
  norm_Fx_force : Scope
  rollAngle : Scope
  sideslip angle : Scope
  sideslip angle1 : Scope
  steering angle : Scope
  total z estimated : Scope
  total z force : Scope
  whl_speed_cog : Scope
  wires:
  [T_req] -> To File1/1, "T_requested "/1
  [Mz_error] -> Mux9/1  "error"
  [Mz_ref] -> Mux9/2  "ref"
  Mux9/1 -> Mz_tracking/1
  Mux5/1 -> effectFL_el1/1, To File4/1
  Mux11/1 -> To File5/1
  Mux12/1 -> To File6/1
  Mux13/1 -> To File7/1
  Subsystem/1(Power debug) -> Bus Selector1/1
  Bus Selector1/1 -> Mux5/1  "<Pm_FL>"
  Bus Selector1/2 -> Gain/1, effectFL_el/1, Mux5/2  "<Pe_FL>"
  Bus Selector1/3 -> Mux11/1  "<Pm_FR>"
  Bus Selector1/4 -> Gain12/1, Mux11/2  "<Pe_FR>"
  Bus Selector1/5 -> Mux12/1  "<Pm_RL>"
  Bus Selector1/6 -> Gain13/1, Mux12/2  "<Pe_RL>"
  Bus Selector1/7 -> Mux13/1  "<Pm_RR>"
  Bus Selector1/8 -> Gain14/1, Mux13/2  "<Pe_RR>"
  whl_speed/1 -> Bus Selector2/1
  Bus Selector2/4 -> Mux14/4  "<RR>"
  Bus Selector2/3 -> Mux14/3  "<RL>"
  Bus Selector2/2 -> Mux14/2  "<FR>"
  Bus Selector2/1 -> Mux14/1  "<FL>"
  Mux14/1 -> whl_speed_cog/1
  Fx_est/1 -> Bus Selector3/1
  Bus Selector3/1 -> Mux15/1  "<FL>"
  Bus Selector3/2 -> Mux15/2  "<FR>"
  Bus Selector3/3 -> Mux15/3  "<RL>"
  Bus Selector3/4 -> Mux15/4  "<RR>"
  Mux15/1 -> Fx_estScope/1
  Read CM Dict53/1 -> Aero_Fx/1  "FL"
  Read CM Dict10/1 -> To File2/1, Rate Transition1/1  "V_x"
  Mux10/1 -> "Vx_ms "/1
  Rate Transition1/1 -> Gain9/1, Mux10/1  "V_x"
  Data Type Conversion1/1 -> Mux10/2  "V_est"
  Gain9/1 -> Mux20/1, Vx_kmh/1
  Mux20/1 -> Aero_Fz/1
  Read CM Dict49/1 -> Rate Transition2/1  "FL"
  Rate Transition2/1 -> Mux20/2
  Gain/1 -> Mux21/1  "Current FL"
  Gain12/1 -> Mux21/2  "Current FR"
  Gain13/1 -> Mux21/3  "Current RL"
  Gain14/1 -> Mux21/4  "Current RR"
  Mux21/1 -> To File9/1
  norm_long_tire_force/1 -> Bus Selector5/1
  Bus Selector5/1 -> Mux22/1  "<FL>"
  Bus Selector5/4 -> Mux22/4  "<RR>"
  Bus Selector5/3 -> Mux22/3  "<RL>"
  Bus Selector5/2 -> Mux22/2  "<FR>"
  Mux22/1 -> norm_Fx_force/1
  Rate Transition3/1 -> Discrete Derivative/1
  Saturation/1 -> Fl_derivate/1
  Abs/1 -> Saturation/1
  Discrete Derivative/1 -> Abs/1
  Mux2/1 -> eng rot/1, To File/1
  Read CM Dict27/1 -> Gain3/1
  Read CM Dict26/1 -> Gain1/1
  Gain15/1 -> Mux2/4  "Motor_RPM"
  Gain3/1 -> Gain15/1
  Gain2/1 -> Mux2/3  "Motor_RPM"
  Gain1/1 -> Gain2/1
  Gain11/1 -> Mux2/2  "Motor_RPM"
  Gain10/1 -> Gain11/1
  Read CM Dict25/1 -> Gain10/1
  Read CM Dict24/1 -> Gain7/1
  Gain4/1 -> Mux2/1, Rate Transition3/1  "Motor_RPM"
  Gain7/1 -> Gain4/1
  Radians to Degrees1/1 -> Mux4/2
  Mux4/1 -> steering angle/1
  Read CM Dict3/1 -> Radians to Degrees/1
  Read CM Dict4/1 -> Radians to Degrees1/1
  Radians to Degrees/1 -> Mux4/1
  Read CM Dict48/1 -> Radians to Degrees7/1
  Radians to Degrees7/1 -> rollAngle/1
  Read CM Dict9/1 -> ay/1
  Read CM Dict8/1 -> ax/1
  Read CM Dict1/1 -> "longSlip "/1
  Mux16/1 -> Fx_CM_scope/1
  Read CM Dict18/1 -> Mux16/2  "Fx_FR"
  Read CM Dict19/1 -> Mux16/4  "Fx_RR"
  Read CM Dict20/1 -> Mux16/3  "Fx_RL"
  Read CM Dict/1 -> Mux16/1  "Fx_FL"
  Mux18/1 -> FY_CM/1
  Read CM Dict22/1 -> Mux18/2  "Fy_FR"
  Read CM Dict5/1 -> Mux18/3  "Fy_RL"
  Read CM Dict23/1 -> Mux18/4  "Fy_RR"
  Read CM Dict21/1 -> Mux18/1  "Fy_FL"
  Data Type Conversion10/1 -> Mux3/3  "RL"
  Data Type Conversion7/1 -> Mux3/2  "FR"
  Mux3/1 -> Rate Transition4/1, Fzi/1
  Read CM Dict7/1 -> Data Type Conversion8/1
  Read CM Dict11/1 -> Data Type Conversion9/1
  Read CM Dict6/1 -> Data Type Conversion7/1
  Data Type Conversion9/1 -> Mux3/4  "RR"
  Read CM Dict28/1 -> Data Type Conversion10/1
  Data Type Conversion8/1 -> Mux3/1  "FL"
  Read CM Dict30/1 -> Mux6/4  "RR"
  Read CM Dict29/1 -> Mux6/3  "RL"
  Read CM Dict32/1 -> Mux6/2  "FR"
  Mux6/1 -> friction coefficients/1
  Read CM Dict31/1 -> Mux6/1  "FL"
  Gain6/1 -> To File3/1
  Gain5/1 -> "Motor Torques "/1
  Read CM Dict43/1 -> Mux8/3  "Mot_RL"
  Read CM Dict44/1 -> Mux8/4  "Mot_RR"
  Read CM Dict41/1 -> Mux8/1  "Mot_FL"
  Mux8/1 -> Gain6/1, Gain5/1
  Read CM Dict42/1 -> Mux8/2  "Mot_FR"
  Mux17/1 -> effRadius/1
  Data Type Conversion6/1 -> Mux17/4  "R_RR"
  Read CM Dict35/1 -> Data Type Conversion6/1
  Read CM Dict34/1 -> Data Type Conversion13/1
  Data Type Conversion13/1 -> Mux17/2  "R_FR"
  Data Type Conversion11/1 -> Mux17/3  "R_RL"
  Data Type Conversion12/1 -> Mux17/1  "R_FL"
  Read CM Dict36/1 -> Data Type Conversion11/1
  Read CM Dict33/1 -> Data Type Conversion12/1
  Read CM Dict38/1 -> Radians to Degrees2/1
  Radians to Degrees2/1 -> sideslip angle/1
  Mux23/1 -> Extract and scale to deg compare to CM output in individual error/1(SA_CM), Slip angles CM/1
  Read CM Dict40/1 -> FR/1  "FR"
  Read CM Dict39/1 -> FL/1  "FL"
  Read CM Dict17/1 -> RR/1  "RL"
  RR/1 -> Mux23/4
  Read CM Dict37/1 -> RL/1  "RL"
  RL/1 -> Mux23/3
  FR/1 -> Mux23/2
  FL/1 -> Mux23/1
  [yaw_rate_ref] -> Data Type Conversion/1, Simulation Results Logging/1(r_ref)  "r_ref"
  Bus Selector4/4 -> Mux19/4  "<RR>"
  Mux19/1 -> SR_i/1, To File8/1
  Bus Selector4/1 -> Mux19/1  "<FL>"
  Bus Selector4/2 -> Mux19/2  "<FR>"
  Bus Selector4/3 -> Mux19/3  "<RL>"
  "SR "/1 -> Simulation Results Logging/2(SR), Bus Selector4/1
  Data Type Conversion/1 -> Mux1/2  "r_ref"
  Rate Transition/1 -> Mux1/1  "r"
  Mux1/1 -> Yaw rate tracking/1
  Read CM Dict2/1 -> Rate Transition/1  "r"
  Subtract/1 -> Fz_error/1
  Bus Selector6/1 -> Mux7/1  "<Fz_FL>"
  Bus Selector6/2 -> Mux7/2  "<Fz_FR>"
  Bus Selector6/3 -> Mux7/3  "<Fz_RL>"
  Bus Selector6/4 -> Mux7/4  "<Fz_RR>"
  Mux7/1 -> Subtract/1, addall1/1(In1)
  Rate Transition4/1 -> Subtract/2, addall/1(In1)
  addall/1(Out1) -> total z force/1, Subtract1/2
  addall1/1(Out1) -> total z estimated/1, Subtract1/1
  Subtract1/1 -> Fz_error total/1
  Read CM Dict12/1 -> "Aero downforce "/1
  DamperRateLookup/1 -> damper force/1  "Fz_damp_FL"
  Bus Selector7/1 -> DamperRateLookup/1  "<damper_rate_FL>"
  Bus Selector7/2 -> DamperRateLookup1/1  "<damper_rate_FR>"
  Bus Selector7/3 -> DamperRateLookup2/1  "<damper_rate_RL>"
  Bus Selector7/4 -> DamperRateLookup3/1  "<damper_rate_RR>"
  DamperRateLookup1/1 -> damper force/2
  DamperRateLookup2/1 -> damper force/3
  DamperRateLookup3/1 -> damper force/4
  Sensors/1 -> [sensor], Bus Selector8/1, Bus Selector7/1  "V_est"
  Constant/1 -> Fz_error/2
  Bus Selector8/1 -> delta SW/1  "<steering_wheel_angle>"
  Read CM Dict13/1 -> Rate Transition5/1
  Rate Transition5/1 -> Sum/1
  Sum/1 -> delta SW/2
  Constant1/1 -> Sum/2
  [states] -> Bus Selector6/1
  states/1 -> [states]
  SA calculation/1(Out1) -> Extract and scale to deg compare to CM output in individual error/2(In1)
  [sensor] -> SA calculation/1(In1)
  Extract and scale to deg compare to CM output in individual error/1(FL) -> SA estimate error/1
  Extract and scale to deg compare to CM output in individual error/2(FR) -> SA estimate error/2
  Extract and scale to deg compare to CM output in individual error/3(RL) -> SA estimate error/3
  Extract and scale to deg compare to CM output in individual error/4(RR) -> SA estimate error/4
  Radians to Degrees3/1 -> FL steer ang lookup deg/1, FR steer ang lookup deg/1
  Degrees to Radians1/1 -> ?
  FR steer ang lookup deg/1 -> Degrees to Radians1/1
  Degrees to Radians/1 -> ?
  FL steer ang lookup deg/1 -> Degrees to Radians/1
  Bus Selector9/1 -> Radians to Degrees3/1  "<steering_wheel_angle>"
  Read CM Dict45/1 -> Radians to Degrees4/1
  Radians to Degrees4/1 -> sideslip angle1/1
  Mux24/1 -> Extract and scale to deg compare to CM output in individual error1/1(SA_CM), Slip ratios CM1/1
  Read CM Dict47/1 -> FR1/1  "FR"
  Read CM Dict46/1 -> FL1/1  "FL"
  Read CM Dict15/1 -> RR1/1  "RL"
  RR1/1 -> Mux24/4
  Read CM Dict16/1 -> RL1/1  "RL"
  RL1/1 -> Mux24/3
  FR1/1 -> Mux24/2
  FL1/1 -> Mux24/1
  Extract and scale to deg compare to CM output in individual error1/1(FL) -> SA estimate error1/1
  Extract and scale to deg compare to CM output in individual error1/2(FR) -> SA estimate error1/2
  Extract and scale to deg compare to CM output in individual error1/3(RL) -> SA estimate error1/3
  Extract and scale to deg compare to CM output in individual error1/4(RR) -> SA estimate error1/4
  Bus Selector10/1 -> Bus Creator/1  "<SR_FL>"
  Bus Selector10/2 -> Bus Creator/2  "<SR_FR>"
  Bus Selector10/3 -> Bus Creator/3  "<SR_RL>"
  Bus Selector10/4 -> Bus Creator/4  "<SR_RR>"
  [states] -> Bus Selector10/1
  Bus Creator/1 -> Extract and scale to deg compare to CM output in individual error1/2(In1)
  TV_monitoring/1 -> Bus Selector12/1
  Bus Selector12/3 -> TV_monitor/1  "<percentage_delivered_torque>"
  Bus Selector12/4 -> [Mz_error]  "<Mz_error>"
  Bus Selector12/5 -> [yaw_rate_ref]  "<yaw_rate_ref>"
  Bus Selector12/6 -> [T_req]  "<T_req>"
  Bus Selector12/7 -> [Mz_ref]  "<Mz_ref>"
  [Mz_ref] -> TV_monitor/2
  [yaw_rate_ref] -> TV_monitor/3
  [T_req] -> TV_monitor/4
  [Mz_error] -> TV_monitor/5
  Read CM Dict50/1 -> To File11/1
  Rate Transition50/1 -> Mux25/1
  Rate Transition49/1 -> Mux25/2
  Rate Transition51/1 -> Mux25/3
  [yaw_rate_ref] -> Rate Transition50/1
  [Mz_error] -> Rate Transition49/1
  [Mz_ref] -> Rate Transition51/1
  Mux25/1 -> To File10/1
  Steering wheel ang-vel2/1 -> Mux26/2
  Steering wheel angle3/1 -> Mux26/3
  Steering wheel ang-vel3/1 -> Mux26/4
  Steering wheel angle2/1 -> Mux26/1
  Mux26/1 -> To File12/1
  Bus Selector12/8 -> [Max_motor_torque]  "<maxMotorTorque>"
  [Max_motor_torque] -> TV_monitor/6
  [Max_motor_torque] -> add_elements/1(In1)
  add_elements/1(Out1) -> TV_monitor/7
  ? -> Bus Selector11/1

== system TV_2017_HIL/CarMaker/DrivMan2 ==
  note: There's rarely a reason to override DrivMan signals.
      | Use the VehicleControl interface for this purpose.
  Sync_In : Inport
  Env.Misc : Inport  Port=2
  BusCreator : BusCreator  Inputs=17
  Demux : Demux  Outputs=17
  DrivMan : S-Function  FunctionName=CM_Sfun  Parameters='DrivMan'  SFunctionDeploymentMode=off  EnableBusSupport=off
  Sync_Out : Outport
  DrivMan.Out : Outport  Port=2
  wires:
  Demux/17 -> BusCreator/17  "DrivMan Steering Trq"
  Demux/16 -> BusCreator/16  "DrivMan Steering AngAcc"
  Demux/15 -> BusCreator/15  "DrivMan Steering AngVel"
  Demux/14 -> BusCreator/14  "DrivMan Steering Ang"
  Demux/13 -> BusCreator/13  "DrivMan Gas"
  Demux/12 -> BusCreator/12  "DrivMan Clutch"
  Demux/11 -> BusCreator/11  "DrivMan BrakePark"
  Demux/10 -> BusCreator/10  "DrivMan Brake"
  Demux/9 -> BusCreator/9  "DrivMan GearNo"
  Demux/8 -> BusCreator/8  "DrivMan SelectorCtrl"
  Demux/7 -> BusCreator/7  "DrivMan UserSignal4"
  Demux/6 -> BusCreator/6  "DrivMan UserSignal3"
  Demux/5 -> BusCreator/5  "DrivMan UserSignal2"
  Demux/4 -> BusCreator/4  "DrivMan UserSignal1"
  Demux/3 -> BusCreator/3  "DrivMan UserSignal0"
  Demux/2 -> BusCreator/2  "DrivMan Key"
  Demux/1 -> BusCreator/1  "DrivMan SST"
  Env.Misc/1 -> DrivMan/2
  Sync_In/1 -> DrivMan/1
  DrivMan/1 -> Sync_Out/1
  BusCreator/1 -> DrivMan.Out/1
  DrivMan/2 -> Demux/1

== system TV_2017_HIL/CarMaker/DrivMan3 ==
  note: There's rarely a reason to override DrivMan signals.
      | Use the VehicleControl interface for this purpose.
  Sync_In : Inport
  Env.Misc : Inport  Port=2
  BusCreator : BusCreator  Inputs=17
  Demux : Demux  Outputs=17
  DrivMan : S-Function  FunctionName=CM_Sfun  Parameters='DrivMan'  SFunctionDeploymentMode=off  EnableBusSupport=off
  Sync_Out : Outport
  DrivMan.Out : Outport  Port=2
  wires:
  Demux/17 -> BusCreator/17  "DrivMan Steering Trq"
  Demux/16 -> BusCreator/16  "DrivMan Steering AngAcc"
  Demux/15 -> BusCreator/15  "DrivMan Steering AngVel"
  Demux/14 -> BusCreator/14  "DrivMan Steering Ang"
  Demux/13 -> BusCreator/13  "DrivMan Gas"
  Demux/12 -> BusCreator/12  "DrivMan Clutch"
  Demux/11 -> BusCreator/11  "DrivMan BrakePark"
  Demux/10 -> BusCreator/10  "DrivMan Brake"
  Demux/9 -> BusCreator/9  "DrivMan GearNo"
  Demux/8 -> BusCreator/8  "DrivMan SelectorCtrl"
  Demux/7 -> BusCreator/7  "DrivMan UserSignal4"
  Demux/6 -> BusCreator/6  "DrivMan UserSignal3"
  Demux/5 -> BusCreator/5  "DrivMan UserSignal2"
  Demux/4 -> BusCreator/4  "DrivMan UserSignal1"
  Demux/3 -> BusCreator/3  "DrivMan UserSignal0"
  Demux/2 -> BusCreator/2  "DrivMan Key"
  Demux/1 -> BusCreator/1  "DrivMan SST"
  Env.Misc/1 -> DrivMan/2
  Sync_In/1 -> DrivMan/1
  DrivMan/1 -> Sync_Out/1
  BusCreator/1 -> DrivMan.Out/1
  DrivMan/2 -> Demux/1
